simulink model "WORKINGFINAL_Neat"  (R2022a)
settings: Solver=FixedStepAuto  StartTime=0.0  StopTime=10.0  RelTol=1e-3  EnableMultiTasking=on
undefined symbols (not defined in the file or in its folder): InputPWM, WheelSpeed
libraries: arduinolib x11, mobileRoboticsTrainingLib x1
settings Model: ExtModeTrigDuration=2  Creator=heath  LastModifiedBy=heath
settings OptimizationCC: EnhancedBackFolding=on  PassReuseOutputArgsAs=Individual arguments  ZeroExternalMemoryAtStartup=off  ZeroInternalMemoryAtStartup=off  MaxStackSize=64  OptimizeBlockOrder=speed  DifferentSizesBufferReuse=on  OptimizationCustomize=off  EfficientTunableParamExpr=on
settings DebuggingCC: MultiTaskDSMMsg=none  ParameterTunabilityLossMsg=error
settings HardwareCC: ProdBitPerPointer=32  ProdBitPerSizeT=32  ProdBitPerPtrDiffT=32  ProdLargestAtomicInteger=Long  ProdLargestAtomicFloat=Double  ProdWordSize=32  ProdHWDeviceType=ARM Compatible->ARM Cortex  UseEmbeddedCoderFeatures=off  UseSimulinkCoderFeatures=off
settings SFSimCC: MATLABDynamicMemAlloc=off
settings RTWCC: SystemTargetFile=ert.tlc  HardwareBoard=Arduino Nano 33 IoT  TemplateMakefile=ert_default_tmf  Toolchain=Arduino ARM  BuildConfiguration=Faster Runs
settings CodeAppCC: ForceParamTrailComments=on  IgnoreCustomStorageClasses=off  OperatorAnnotations=on  SimulinkDataObjDesc=on  SFDataObjDesc=on  InsertBlockDesc=on
settings ERTTargetCC: SupportContinuousTime=on  SupportNonInlinedSFcns=on  SupportVariableSizeSignals=on  ExtModeTransport=3  ExtModeStaticAlloc=on  ExtModeStaticAllocSize=8192  ExtModeMexFile=ext_xcp  ExtModeIntrfLevel=Level2 - Open

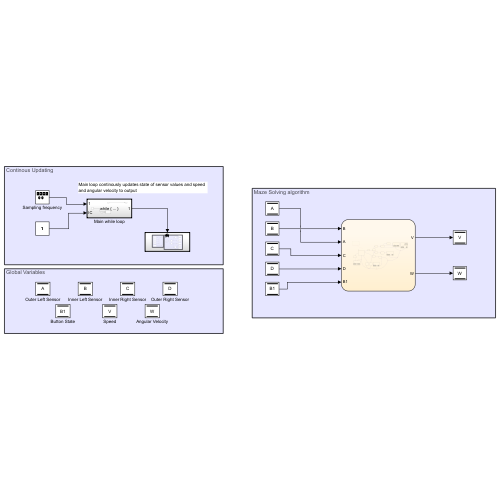
[thumbnail: Simulink's stored preview of the top-level diagram]
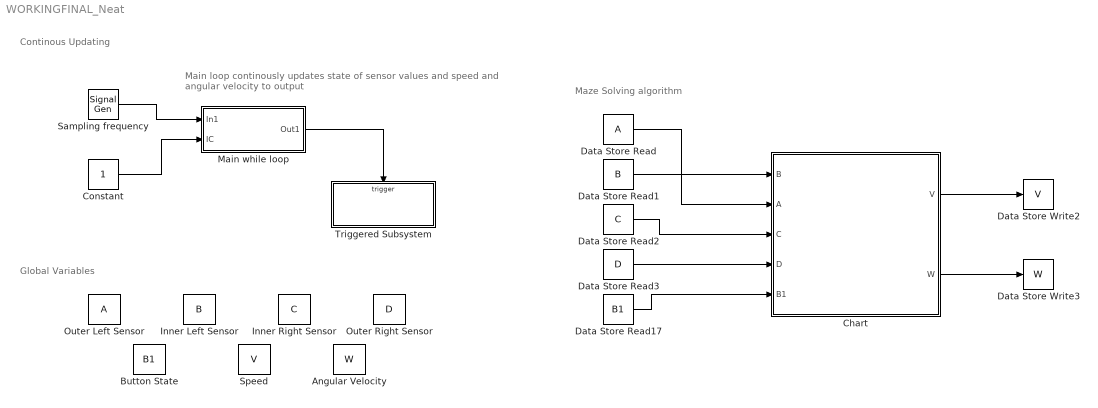
== system WORKINGFINAL_Neat ==
  note: Maze Solving algorithm
  note: Global Variables
  note: Continous Updating
  note: Main loop continously updates state of sensor values and speed and angular velocity to output
  Angular Velocity : DataStoreMemory  DataStoreName=W  WriteAfterWriteMsg=warning  ShowAdditionalParam=off
  Button State : DataStoreMemory  DataStoreName=B1  WriteAfterWriteMsg=warning  ShowAdditionalParam=off
  Chart : Stateflow chart  TreatAsAtomicUnit=on
  Constant : Constant
  Data Store Read : DataStoreRead  IndexOptions=Index vector (dialog)  Indices=1  OutputSizes=1
  Data Store Read1 : DataStoreRead  DataStoreName=B  IndexOptions=Index vector (dialog)  Indices=1  OutputSizes=1
  Data Store Read17 : DataStoreRead  DataStoreName=B1  IndexOptions=Index vector (dialog)  Indices=1  OutputSizes=1
  Data Store Read2 : DataStoreRead  DataStoreName=C  IndexOptions=Index vector (dialog)  Indices=1  OutputSizes=1
  Data Store Read3 : DataStoreRead  DataStoreName=D  IndexOptions=Index vector (dialog)  Indices=1  OutputSizes=1
  Data Store Write2 : DataStoreWrite  DataStoreName=V  IndexOptions=Index vector (dialog)  Indices=1  OutputSizes=1
  Data Store Write3 : DataStoreWrite  DataStoreName=W  IndexOptions=Index vector (dialog)  Indices=1  OutputSizes=1
  Inner Left Sensor : DataStoreMemory  DataStoreName=B  WriteAfterWriteMsg=warning  ShowAdditionalParam=off
  Inner Right Sensor : DataStoreMemory  DataStoreName=C  WriteAfterWriteMsg=warning  ShowAdditionalParam=off
  Main while loop : Subsystem  TreatAsAtomicUnit=on
  Outer Left Sensor : DataStoreMemory  WriteAfterWriteMsg=warning  ShowAdditionalParam=off
  Outer Right Sensor : DataStoreMemory  DataStoreName=D  WriteAfterWriteMsg=warning  ShowAdditionalParam=off
  Sampling frequency : SignalGenerator  WaveForm=square  Frequency=100
  Speed : DataStoreMemory  DataStoreName=V  WriteAfterWriteMsg=warning  ShowAdditionalParam=off
  Triggered Subsystem : Subsystem  TreatAsAtomicUnit=on
  wires:
  Sampling frequency/1 -> Main while loop/1(In1)
  Constant/1 -> Main while loop/2(IC)
  Main while loop/1(Out1) -> Triggered Subsystem/Trigger
  Chart/1(V) -> Data Store Write2/1
  Data Store Read3/1 -> Chart/4(D)
  Data Store Read2/1 -> Chart/3(C)
  Data Store Read1/1 -> Chart/1(B)
  Chart/2(W) -> Data Store Write3/1
  Data Store Read/1 -> Chart/2(A)
  Data Store Read17/1 -> Chart/5(B1)

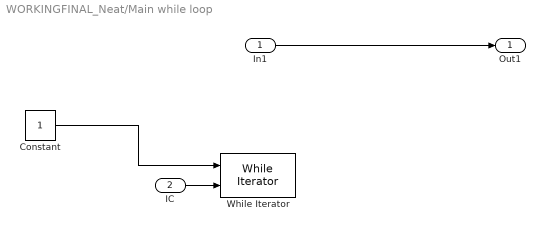
== system WORKINGFINAL_Neat/Main while loop ==
  In1 : Inport
  IC : Inport  Port=2
  Constant : Constant
  While Iterator : WhileIterator
  Out1 : Outport
  wires:
  IC/1 -> While Iterator/2
  In1/1 -> Out1/1
  Constant/1 -> While Iterator/1

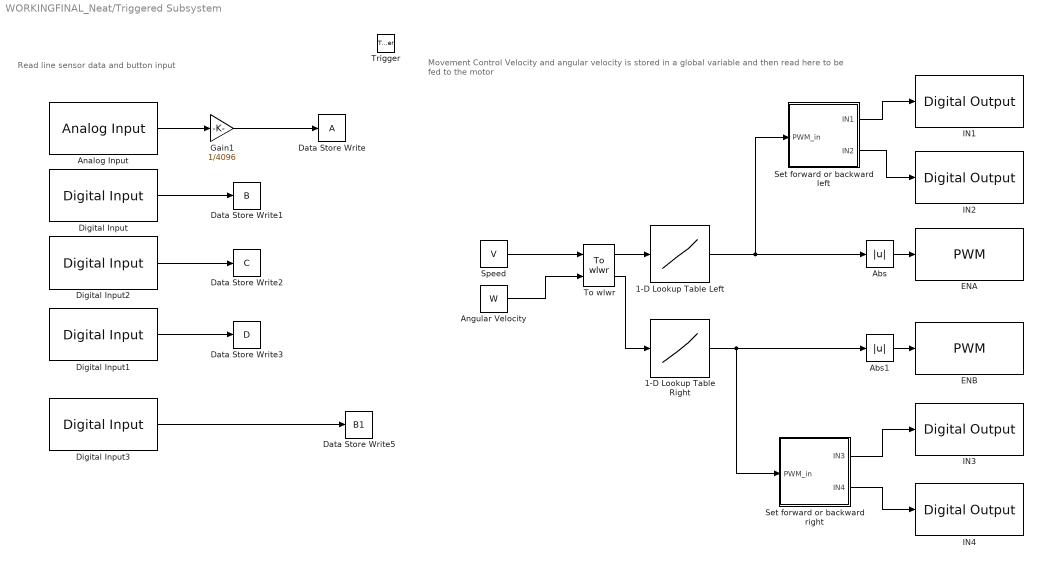
== system WORKINGFINAL_Neat/Triggered Subsystem ==
  note: Read line sensor data and button input
  note: Movement Control
      | Velocity and angular velocity is stored in a global variable and then read here to be fed to the motor
  Trigger : TriggerPort  TriggerType=either  VariantControl=(inherit)
  1-D Lookup Table Left : Lookup_n-D  NumberOfTableDimensions=1  BreakpointsForDimension1=WheelSpeed  Table=InputPWM  InternalRulePriority=Speed  RndMeth=Simplest
  1-D Lookup Table Right : Lookup_n-D  NumberOfTableDimensions=1  BreakpointsForDimension1=WheelSpeed  Table=InputPWM  InternalRulePriority=Speed  RndMeth=Simplest
  Abs : Abs  SaturateOnIntegerOverflow=off
  Abs1 : Abs  SaturateOnIntegerOverflow=off
  Analog Input : arduinolib/Analog Input  pinNumber=0  ReadResultsOnly=off  ConversionTriggerSource=Software  ExternalTriggerType=uint32( 0 )  OutputDataType=uint16  EnableConversionCompleteNotify=off  EnableOuputStatus=off  SampleTime=-1  blockPlatform=arduino
  Angular Velocity : DataStoreRead  DataStoreName=W  IndexOptions=Index vector (dialog)  Indices=1  OutputSizes=1
  Data Store Write : DataStoreWrite  IndexOptions=Index vector (dialog)  Indices=1  OutputSizes=1
  Data Store Write1 : DataStoreWrite  DataStoreName=B  IndexOptions=Index vector (dialog)  Indices=1  OutputSizes=1
  Data Store Write2 : DataStoreWrite  DataStoreName=C  IndexOptions=Index vector (dialog)  Indices=1  OutputSizes=1
  Data Store Write3 : DataStoreWrite  DataStoreName=D  IndexOptions=Index vector (dialog)  Indices=1  OutputSizes=1
  Data Store Write5 : DataStoreWrite  DataStoreName=B1  IndexOptions=Index vector (dialog)  Indices=1  OutputSizes=1
  Digital Input : arduinolib/Digital Input  pinNumber=12  mode=Default  Direction=input  SampleTime=-1  blockPlatform=arduino
  Digital Input1 : arduinolib/Digital Input  pinNumber=8  mode=Default  Direction=input  SampleTime=-1  blockPlatform=arduino
  Digital Input2 : arduinolib/Digital Input  pinNumber=11  mode=Default  Direction=input  SampleTime=-1  blockPlatform=arduino
  Digital Input3 : arduinolib/Digital Input  pinNumber=13  mode=Default  Direction=input  SampleTime=-1  blockPlatform=arduino
  ENA : arduinolib/PWM  pinNumber=3  frequencyType=Default  desiredFrequency=490.2  achievableFrequency=490.2
  ENB : arduinolib/PWM  pinNumber=2  frequencyType=Default  desiredFrequency=490.2  achievableFrequency=490.2
  Gain1 : Gain  Gain=1/4096
  IN1 : arduinolib/Digital Output  pinNumber=4  Direction=output  blockPlatform=arduino
  IN2 : arduinolib/Digital Output  pinNumber=5  Direction=output  blockPlatform=arduino
  IN3 : arduinolib/Digital Output  pinNumber=6  Direction=output  blockPlatform=arduino
  IN4 : arduinolib/Digital Output  pinNumber=7  Direction=output  blockPlatform=arduino
  Set forward or backward left : Stateflow chart  TreatAsAtomicUnit=on
  Set forward or backward right : Stateflow chart  TreatAsAtomicUnit=on
  Speed : DataStoreRead  DataStoreName=V  IndexOptions=Index vector (dialog)  Indices=1  OutputSizes=1
  To wlwr : mobileRoboticsTrainingLib/To wlwr  axleLength=axleLength  wheelR=wheelR
  wires:
  Set forward or backward right/2(IN4) -> IN4/1
  Set forward or backward left/2(IN2) -> IN2/1
  Set forward or backward left/1(IN1) -> IN1/1
  Abs1/1 -> ENB/1
  Abs/1 -> ENA/1
  1-D Lookup Table Right/1 -> Set forward or backward right/1(PWM_in), Abs1/1
  Set forward or backward right/1(IN3) -> IN3/1
  To wlwr/2 -> 1-D Lookup Table Right/1
  To wlwr/1 -> 1-D Lookup Table Left/1
  1-D Lookup Table Left/1 -> Set forward or backward left/1(PWM_in), Abs/1
  Speed/1 -> To wlwr/1
  Angular Velocity/1 -> To wlwr/2
  Analog Input/1 -> Gain1/1
  Digital Input/1 -> Data Store Write1/1
  Digital Input2/1 -> Data Store Write2/1
  Digital Input1/1 -> Data Store Write3/1
  Gain1/1 -> Data Store Write/1
  Digital Input3/1 -> Data Store Write5/1

== stateflow chart WORKINGFINAL_Neat/Chart ==
  settings: updateMethod=CONTINUOUS
  state Initial [commented out]
    entry:
    W = 0;
    V = 0;
    %LEDController.SetLEDState(LEDStates.IDLE);
  state Stop
    entry:
    done=0;
    V = 0;
    W = 0;
  state Find_Line
    entry:
    done = 0;
    state Found
      entry:
      done=1;
    state Finding_line
      entry:
      V=0.13;
    (default) -> Finding_line
    Finding_line -> Found : [B<0.5||C<0.5]
  state Turn_left_90_junc
    entry:
    done = 0;
    state PassLineDelay
      entry:
      V=0;
      W=1.5;
    state Turn
      entry:
      V=0;
      W = 1.5;
    state Stop
      entry:
      done=1;
    (default) -> PassLineDelay
    PassLineDelay -> Turn_left_90_junc.Turn : [after(0.5,sec)]
    Turn_left_90_junc.Turn -> Turn_left_90_junc.Stop : [B<0.5]
  state WhereWeAt2
    entry:
    done = 1;
    V=0.13;
  state Delay1
    entry:
    V=0.13;
  state WhereWeAt
    entry:
    V=0.13;
    done=1;
  state Delay0
    entry:
    V=0.13;
  state Follow_Line
    entry:
    V=0.13;
    W=0;
    done=0;
  state Turn_left_90
    entry:
    done = 0;
    state Turn
      entry:
      V=0;
      W = 1.5;
    state Stop
      entry:
      done=1;
    (default) -> Turn_left_90.Turn
    Turn_left_90.Turn -> Turn_left_90.Stop : [B<0.5]
  state Delay2
    entry:
    V=0.13;
  state WhereWeAt3
    entry:
    done = 1;
    V=0.13;
  state Delay3
    entry:
    V=0.13;
  state Delay_180
    entry:
    V=0.13;
  state WhereWeAt4
    entry:
    done = 1;
    V=0.13;
  state Turn_180
    entry:
    done = 0;
    state Turn
      entry:
      V=0;
      W = 1.5;
    state Stop
      entry:
      done=1;
    (default) -> Turn_180.Turn
    Turn_180.Turn -> Turn_180.Stop : [B<0.5]
  state Turn_left
    entry:
    done=0;
    V = 0.13;
    W = 1.5;
    done=1;
  state Turn_right
    entry:
    done=0;
    V = 0.13;
    W = -1.5;
    done=1;
  state Turn_Right_90
    entry:
    done = 0;
    state Turn
      entry:
      V=0;
      W = -1.5;
    state Stop
      entry:
      done=1;
    (default) -> Turn_Right_90.Turn
    Turn_Right_90.Turn -> Turn_Right_90.Stop : [C<0.5]
  WhereWeAt2 -> Stop [order 1] : [A<0.5&&B<0.5&&C<0.5&&D<0.5&&done==1]
  Initial -> ? [commented out] : [B1 > 0.5]
  WhereWeAt2 -> Find_Line [order 2] : [A>0.5&&B>0.5&&C>0.5&&D>0.5&&done==1]
  WhereWeAt -> Delay1 [order 2] : [A<0.5&&D<0.5&&done==1]
  Delay1 -> WhereWeAt2 : [after(0.3,sec)]
  Find_Line -> (junction 206) : [done==1]
  WhereWeAt2 -> Turn_left_90_junc [order 3] : [done==1]
  Turn_left_90_junc -> (junction 206) : [done==1]
  (default) -> Follow_Line
  Follow_Line -> Delay0 [order 3] : [A<0.5||D<0.5]
  Delay0 -> WhereWeAt : [after(0.1,sec)]
  (junction 206) -> (junction 207)
  WhereWeAt -> Delay3 [order 1] : [A>0.5&&D<0.5&&done==1]
  WhereWeAt -> Delay2 [order 3] : [A<0.5&&D>0.5&&done==1]
  WhereWeAt3 -> Turn_left_90 : [done==1]
  Follow_Line -> Turn_right [order 1] : [B<0.5&&C>0.5]
  Delay2 -> WhereWeAt3 : [after(0.3,sec)]
  Follow_Line -> Delay_180 [order 4] : [A>0.5&&B>0.5&&C>0.5&&D>0.5]
  Follow_Line -> Turn_left [order 2] : [B>0.5&&C<0.5]
  (junction 216) -> Follow_Line
  Turn_left_90 -> (junction 207) : [done==1]
  Delay3 -> WhereWeAt4 : [after(0.3,sec)]
  WhereWeAt4 -> (junction 210) [order 1] : [B<0.5&&C<0.5&&done==1]
  (junction 207) -> (junction 210)
  Delay_180 -> Turn_180 : [after(0.3,sec)]
  WhereWeAt4 -> Turn_Right_90 [order 2] : [B>0.5&&C>0.5&&done==1]
  Turn_180 -> (junction 216) : [done==1]
  (junction 214) -> (junction 216)
  (junction 210) -> (junction 212)
  Turn_left -> (junction 214) : [done==1]
  Turn_right -> (junction 214) : [done==1]
  Turn_Right_90 -> (junction 212) : [done==1]
  (junction 212) -> (junction 214)
  data: B input; A input; C input; D input; V output; W output; done local; B1 input

== stateflow chart WORKINGFINAL_Neat/Triggered Subsystem/Set forward or backward left ==
  state Forward
    entry:
    IN1 = 1;
    IN2 = 0;
  state Back
    entry:
    IN1 = 0;
    IN2 = 1;
  (default) -> Forward
  Forward -> Back : [PWM_in<0]
  Back -> Forward : [PWM_in>=0]
  data: PWM_in input; IN1 output; IN2 output

== stateflow chart WORKINGFINAL_Neat/Triggered Subsystem/Set forward or backward right ==
  state Forward
    entry:
    IN4 = 0;
    IN3 = 1;
  state Back
    entry:
    IN4 = 1;
    IN3 = 0;
  (default) -> Forward
  Forward -> Back : [PWM_in<0]
  Back -> Forward : [PWM_in>=0]
  data: PWM_in input; IN3 output; IN4 output
